simulink subsystem "Feedforward_input_interface"  (R2024b)
settings: Solver=VariableStepAuto  StartTime=0.0  StopTime=10.0  RelTol=1e-3
undefined symbols (not defined in the file or in its folder): rpm2rads
settings Model: Creator=Riccardo Grosso  LastModifiedBy=Buton

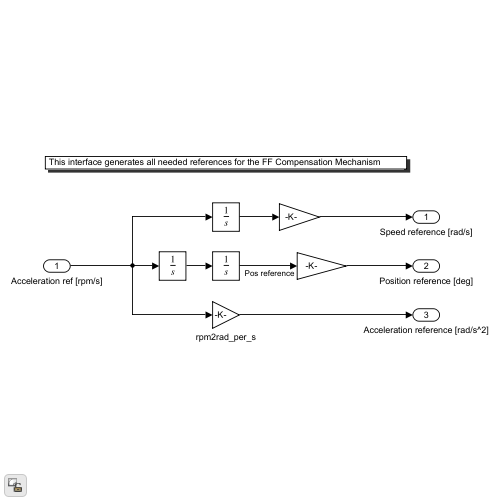
[thumbnail: Simulink's stored preview of the top-level diagram]
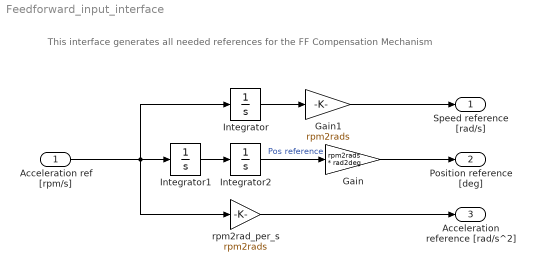
== system Feedforward_input_interface ==
  note: This interface generates all needed references for the FF Compensation Mechanism
  Acceleration ref [rpm/s] : Inport
  Gain : Gain  Gain=rpm2rads * rad2deg
  Gain1 : Gain  Gain=rpm2rads
  Integrator : Integrator
  Integrator1 : Integrator
  Integrator2 : Integrator
  rpm2rad_per_s : Gain  Gain=rpm2rads
  Speed reference [rad/s] : Outport
  Position reference [deg] : Outport  Port=2
  Acceleration reference [rad/s^2] : Outport  Port=3
  wires:
  Integrator2/1 -> Gain/1  "Pos reference"
  Gain1/1 -> Speed reference [rad/s]/1
  Integrator1/1 -> Integrator2/1
  Integrator/1 -> Gain1/1
  Gain/1 -> Position reference [deg]/1
  Acceleration ref [rpm/s]/1 -> rpm2rad_per_s/1, Integrator1/1, Integrator/1
  rpm2rad_per_s/1 -> Acceleration reference [rad/s^2]/1
